simulink model "manchester_receiver"  (R2025a)
settings: Solver=FixedStepDiscrete  StartTime=0.0  StopTime=sim_time  FixedStep=1/fs  RelTol=1e-3
values from neighbouring files (symbols this model uses):
  fs = 8000    [init_receiver.m]    (also in tx_signal.m; tx_workspace.mat)
  KEY = uint8([0x3A, 0x5C, 0x77, 0xC1])    [init_receiver.m]    (also in tx_signal.m = uint8([0x3A,0x5C,0x77,0xC1]))
settings Model: Creator=Subham Sarkar  LastModifiedBy=Subham Sarkar

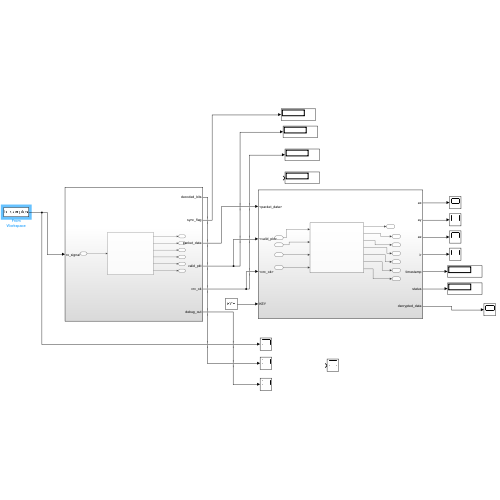
[thumbnail: Simulink's stored preview of the top-level diagram]
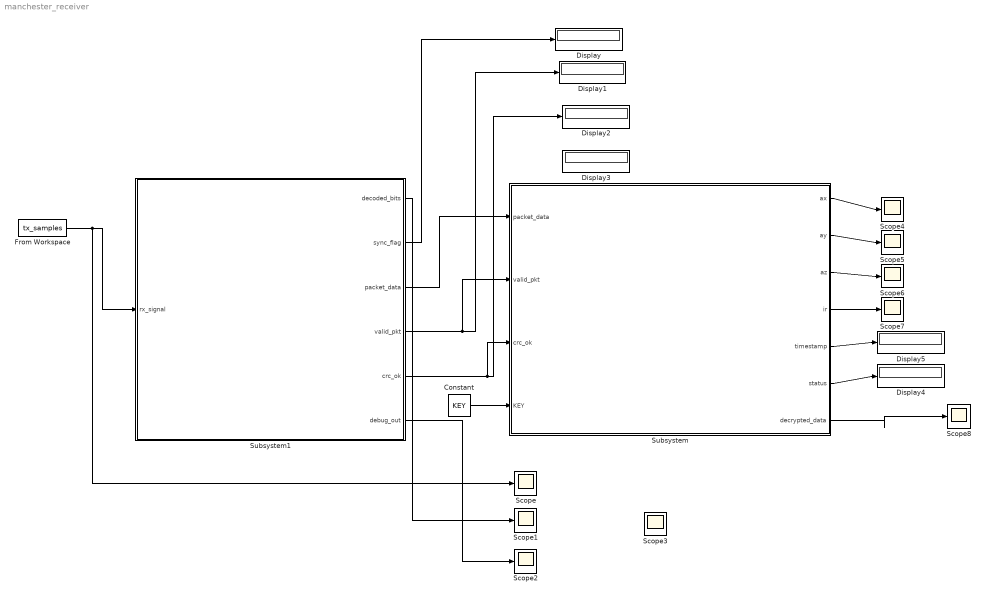
== system manchester_receiver ==
  Constant : Constant  Value=KEY  OutDataTypeStr=uint8
  Display{,1..5} (6 alike) : Display
  From Workspace : FromWorkspace  VariableName=tx_samples  OutDataTypeStr=double  SampleTime=1/fs
  Scope{,1..8} (9 alike) : Scope
      Scope2 settings: DataLoggingVariableName=ScopeData2
      Scope3 settings: DataLoggingVariableName=ScopeData3
      Scope4 settings: DataLoggingVariableName=ScopeData4
      Scope5 settings: DataLoggingVariableName=ScopeData5
      Scope6 settings: DataLoggingVariableName=ScopeData6
      Scope7 settings: DataLoggingVariableName=ScopeData7
      Scope8 settings: DataLoggingVariableName=ScopeData8
  Subsystem : Subsystem
  Subsystem1 : Subsystem
  wires:
  Subsystem1/4(valid_pkt) -> Display1/1, Subsystem/2(valid_pkt)
  Subsystem1/3(packet_data) -> Subsystem/1(packet_data)
  Subsystem1/5(crc_ok) -> Display2/1, Subsystem/3(crc_ok)
  Subsystem1/2(sync_flag) -> Display/1
  From Workspace/1 -> Scope/1, Subsystem1/1(rx_signal)
  Constant/1 -> Subsystem/4(KEY)
  Subsystem1/1(decoded_bits) -> Scope1/1
  Subsystem1/6(debug_out) -> Scope2/1
  Subsystem/1(ax) -> Scope4/1
  Subsystem/2(ay) -> Scope5/1
  Subsystem/3(az) -> Scope6/1
  Subsystem/4(ir) -> Scope7/1
  Subsystem/6(status) -> Display4/1
  Subsystem/5(timestamp) -> Display5/1
  Subsystem/7(decrypted_data) -> Scope8/1

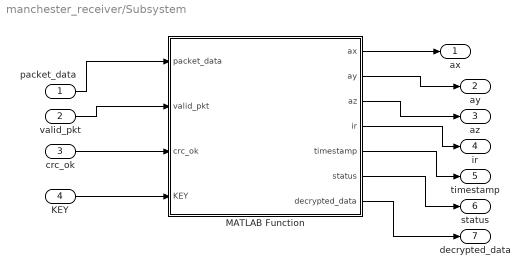
== system manchester_receiver/Subsystem ==
  packet_data : Inport
  valid_pkt : Inport  Port=2
  crc_ok : Inport  Port=3
  KEY : Inport  Port=4
  MATLAB Function : MATLAB Function  TreatAsAtomicUnit=on
  ax : Outport
  ay : Outport  Port=2
  az : Outport  Port=3
  ir : Outport  Port=4
  timestamp : Outport  Port=5
  status : Outport  Port=6
  decrypted_data : Outport  Port=7
  wires:
  packet_data/1 -> MATLAB Function/1(packet_data)
  valid_pkt/1 -> MATLAB Function/2(valid_pkt)
  crc_ok/1 -> MATLAB Function/3(crc_ok)
  KEY/1 -> MATLAB Function/4(KEY)
  MATLAB Function/1(ax) -> ax/1
  MATLAB Function/2(ay) -> ay/1
  MATLAB Function/3(az) -> az/1
  MATLAB Function/4(ir) -> ir/1
  MATLAB Function/5(timestamp) -> timestamp/1
  MATLAB Function/6(status) -> status/1
  MATLAB Function/7(decrypted_data) -> decrypted_data/1

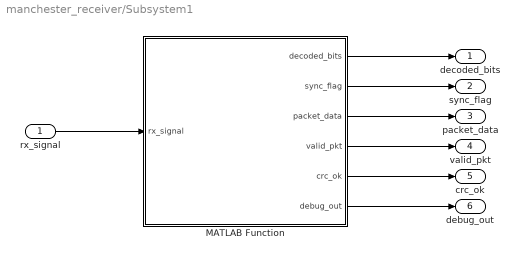
== system manchester_receiver/Subsystem1 ==
  rx_signal : Inport
  MATLAB Function : MATLAB Function  TreatAsAtomicUnit=on
  decoded_bits : Outport
  sync_flag : Outport  Port=2
  packet_data : Outport  Port=3
  valid_pkt : Outport  Port=4
  crc_ok : Outport  Port=5
  debug_out : Outport  Port=6
  wires:
  rx_signal/1 -> MATLAB Function/1(rx_signal)
  MATLAB Function/1(decoded_bits) -> decoded_bits/1
  MATLAB Function/2(sync_flag) -> sync_flag/1
  MATLAB Function/3(packet_data) -> packet_data/1
  MATLAB Function/4(valid_pkt) -> valid_pkt/1
  MATLAB Function/5(crc_ok) -> crc_ok/1
  MATLAB Function/6(debug_out) -> debug_out/1

== matlab function manchester_receiver/Subsystem/MATLAB Function ==
  data: packet_data input; ax output; valid_pkt input; crc_ok input; KEY input; ay output; az output; ir output; timestamp output; status output; decrypted_data output
function [ax, ay, az, ir, timestamp, status, decrypted_data] = packet_processor_block(packet_data, valid_pkt, crc_ok, KEY)
%#codegen
[ax, ay, az, ir, timestamp, decrypted_data] = process_esp32_packet(packet_data, valid_pkt, crc_ok, KEY);
status = valid_pkt && crc_ok;
end

== matlab function manchester_receiver/Subsystem1/MATLAB Function ==
  data: rx_signal input; decoded_bits output; sync_flag output; packet_data output; valid_pkt output; crc_ok output; debug_out output
function [decoded_bits, sync_flag, packet_data, valid_pkt, crc_ok, debug_out] = manchester_decoder_block(rx_signal)
%#codegen
[decoded_bits, sync_flag, packet_data, valid_pkt, crc_ok, debug] = manchester_decoder(rx_signal);
debug_out = [double(debug.man_buf), double(debug.bit_val), double(debug.sync_match)];
end
